simulink model "foc_caller_smoke_autogen"  (R2024a)
settings: Solver=FixedStepDiscrete  StartTime=0.0  StopTime=0.02  FixedStep=5e-5  RelTol=1e-3
settings Model: Creator=黄钟锐  LastModifiedBy=黄钟锐
settings SFSimCC: SimCustomHeaderCode="#include \"sim/foc_sim.h\""
settings SFSimCC: SimUserSources=|
  | src\sim\foc_sim.c
  | src\control\current_controller.c
  | src\control\velocity_controller.c
  | src\foc\foc_math.c
  | src\foc\svpwm.c
settings SFSimCC: SimUserIncludeDirs=|
  | include
  | src
  | src\sim
  | src\control
  | src\foc

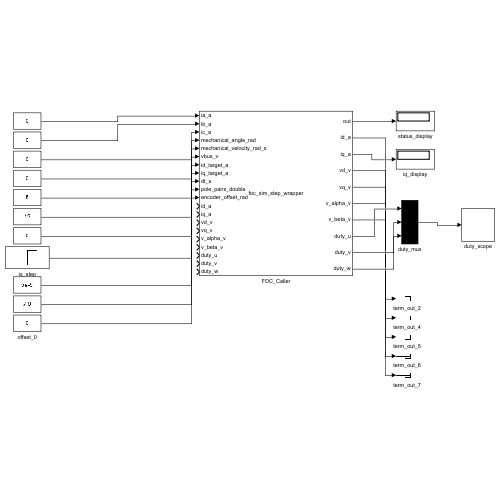
[thumbnail: Simulink's stored preview of the top-level diagram]
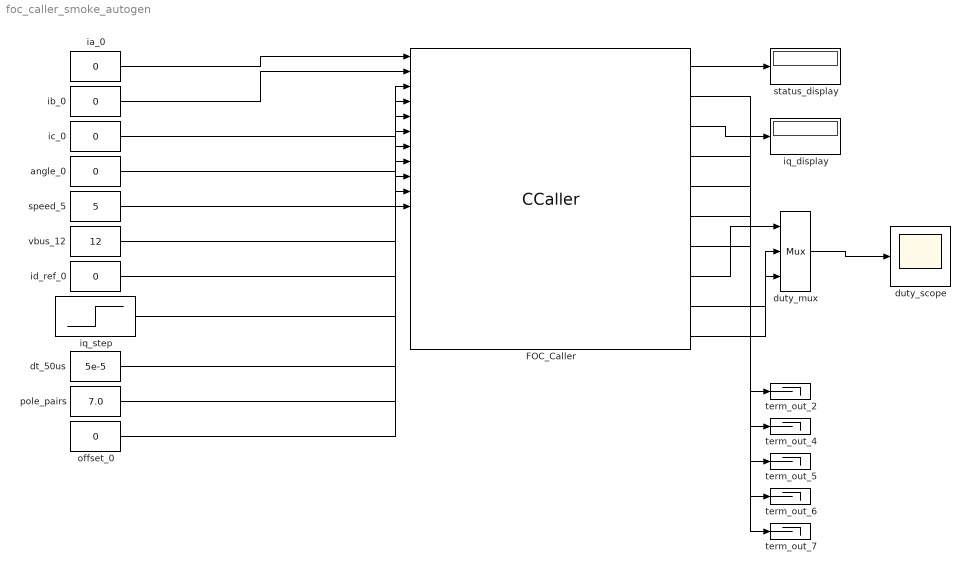
== system foc_caller_smoke_autogen ==
  FOC_Caller : CCaller  FunctionName=foc_sim_step_wrapper  PortSpecificationStruct="%)30     .    8\"0   8    (     @         %    \"    !4    !     0         %  0 \"0    $    _    07)G3F%M90  4&]R=$YA;64 4V-O<&4     26YD97@     5'EP90      4VEZ90      27-';&]B86P   X    P    !@    @    $          4    (     0    ,    !         !   P!O=70 #@   #     &    \"     0         !0    @    !     P    $         $  # &]U=  .    .     8    (    !          %    \"     $    &     0         0  ...(+12198 chars)"  SampleTime=5e-5
  angle_0 : Constant  Value=0  SampleTime=5e-5
  dt_50us : Constant  Value=5e-5  SampleTime=5e-5
  duty_mux : Mux  Inputs=3
  duty_scope : Scope
  ia_0 : Constant  Value=0  SampleTime=5e-5
  ib_0 : Constant  Value=0  SampleTime=5e-5
  ic_0 : Constant  Value=0  SampleTime=5e-5
  id_ref_0 : Constant  Value=0  SampleTime=5e-5
  iq_display : Display
  iq_step : Step  Time=0.005  After=0.5  SampleTime=5e-5
  offset_0 : Constant  Value=0  SampleTime=5e-5
  pole_pairs : Constant  Value=7.0  SampleTime=5e-5
  speed_5 : Constant  Value=5  SampleTime=5e-5
  status_display : Display
  term_out_{2,4..7} (5 alike) : Terminator
  vbus_12 : Constant  Value=12  SampleTime=5e-5
  wires:
  ia_0/1 -> FOC_Caller/1
  ib_0/1 -> FOC_Caller/2
  ic_0/1 -> FOC_Caller/3
  angle_0/1 -> FOC_Caller/4
  speed_5/1 -> FOC_Caller/5
  vbus_12/1 -> FOC_Caller/6
  id_ref_0/1 -> FOC_Caller/7
  iq_step/1 -> FOC_Caller/8
  dt_50us/1 -> FOC_Caller/9
  pole_pairs/1 -> FOC_Caller/10
  offset_0/1 -> FOC_Caller/11
  FOC_Caller/1 -> status_display/1
  FOC_Caller/3 -> iq_display/1
  FOC_Caller/8 -> duty_mux/1
  FOC_Caller/9 -> duty_mux/2
  FOC_Caller/10 -> duty_mux/3
  duty_mux/1 -> duty_scope/1
  FOC_Caller/2 -> term_out_2/1
  FOC_Caller/4 -> term_out_4/1
  FOC_Caller/5 -> term_out_5/1
  FOC_Caller/6 -> term_out_6/1
  FOC_Caller/7 -> term_out_7/1
